simulink library "rtwvariantslib"  (Simulink 7.6)
settings: Solver=FixedStepDiscrete  StartTime=0.0  StopTime=10.0  RelTol=1e-3
undefined symbols (not defined in the file or in its folder): Variant1, Variant2
libraries: rtwvariantslib x2
settings Model: Creator=The MathWorks Inc.

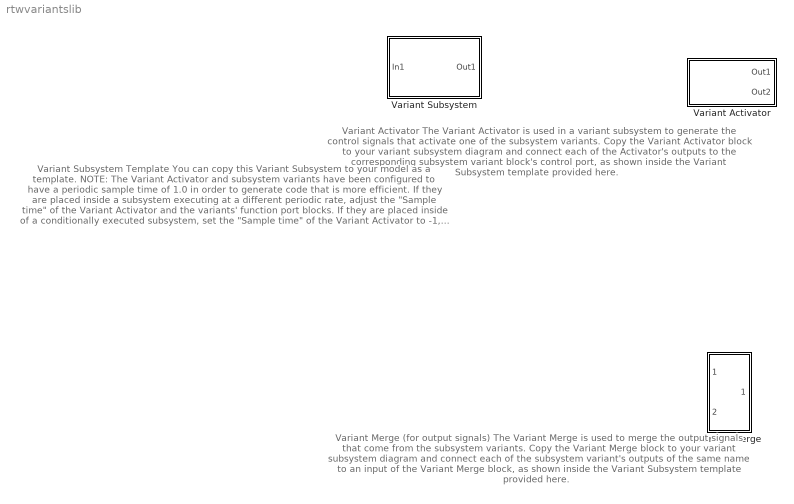
== system rtwvariantslib ==
  note: Variant Merge (for output signals)
      |
      | The Variant Merge
      | is used to merge
      | the output signals
      | that come from the
      | subsystem variants.
      |
      |
      | Copy the Variant Merge block to your
      | variant subsystem diagram and connect
      | each of the subsystem variant's outputs
      | of the same name to an input of
      | the Variant Merge block, as shown
      | inside the Variant Subsystem
      | template provided here.
  note: Variant Activator
      |
      | The Variant Activator
      | is used in a variant
      | subsystem to
      | generate the control
      | signals that activate
      | one of the subsystem
      | variants.
      |
      | Copy the Variant Activator block to your
      | variant subsystem diagram and connect
      | each of the Activator's outputs to
      | the corresponding subsystem
      | variant block's control port, as shown
      | inside the Variant Subsystem
      | template provided here.
  note: Variant Subsystem Template
      |
      | You can copy this
      | Variant Subsystem
      | to your model as a
      | template.
      |
      | NOTE: The Variant Activator and subsystem
      | variants have been configured to have a
      | periodic sample time of 1.0 in order to
      | generate code that is more efficient.
      | If they are placed inside a subsystem
      | executing at a different periodic rate,
      | adjust the "Sample time" of the Variant
      | Activator and the variants' function port
      | blocks.
      | If they are placed inside of a conditionally
      | executed subsystem, set the "Sample time"
      | of the Variant Activator to -1, and the
      | "Sample time type" of the variants' function
      | port blocks to "triggered".
  Variant Activator : Subsystem  mask(Variant Activator){sample_time=1, condition=Variant1,Variant2, gen_preproc_cond=on}
      mask prompts: sample_time "Sample time:"; condition "Variants (comma-separated list of Simulink.Variant objects):"; gen_preproc_cond "Generate preprocessor conditionals"
      mask help:
      | The Variant Activator is used to generate the control signals that activate one of the function-call subsystems.
      |
      | Enter the names of the Variant Objects in the Variants field as a comma-separated list. Variant objects are created in the base workspace and have conditions to determine which variant is active. For example:
      | >>  Variant1 = Simulink.Variant('A==1')
      | >>  Variant2 = Simulink.Variant('A==2')
      | Variant1 is active when A is equal to 1 and Variant2 is active when A is equal to 2. Only one Variant Object can be active during simulation.
      mask init:
      | rtwprivate('VariantActivatorInitializationCommands',condition);
      mask Display: port_label('output',1,'Variant1'); port_label('output',2,'Variant2');
  Variant Merge : Subsystem  mask(Variant Merge){numInputs=2}
      mask prompts: numInputs "Number of Inputs:"
      mask help: This block is used in a variant subsystem to merge the corresponding outputs from subsystem variant blocks.
      mask init:
      | rtwprivate('VariantMergeInitializationCommands',numInputs);
      mask Display: disp('Variant\nMerge')
  Variant Subsystem : Subsystem
      settings: CopyFcn=|
      | set_param(gcb, 'LinkStatus', 'none');
      | set_param(gcb, 'CopyFcn', '');

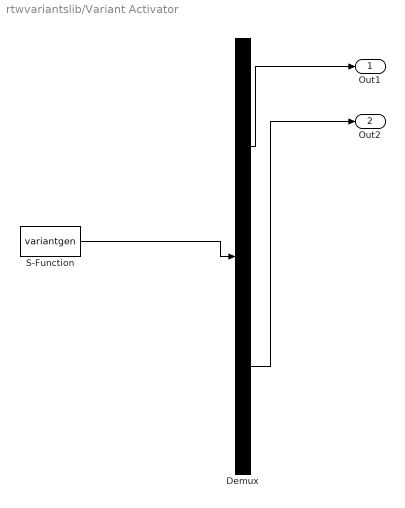
== system rtwvariantslib/Variant Activator ==
  Demux : Demux  Outputs=2
  S-Function : S-Function  FunctionName=variantgen  Parameters=sample_time,1,condition,gen_preproc_cond  EnableBusSupport=off
  Out1 : Outport
  Out2 : Outport  Port=2
  wires:
  Demux/1 -> Out1/1
  S-Function/1 -> Demux/1
  Demux/2 -> Out2/1

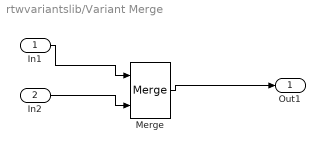
== system rtwvariantslib/Variant Merge ==
  In1 : Inport
  In2 : Inport  Port=2
  Merge : Merge
  Out1 : Outport
  wires:
  In2/1 -> Merge/2
  In1/1 -> Merge/1
  Merge/1 -> Out1/1

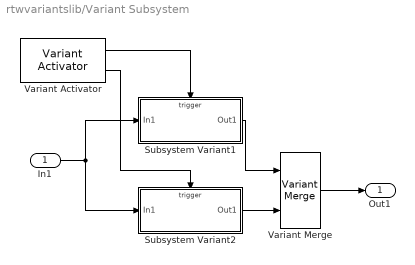
== system rtwvariantslib/Variant Subsystem ==
  In1 : Inport
  Subsystem Variant1 : Subsystem  TreatAsAtomicUnit=on
      settings: CopyFcn=|
      | set_param(gcb, 'LinkStatus', 'none');
      | set_param(gcb, 'CopyFcn', '');
  Subsystem Variant2 : Subsystem  TreatAsAtomicUnit=on
      settings: CopyFcn=|
      | set_param(gcb, 'LinkStatus', 'none');
      | set_param(gcb, 'CopyFcn', '');
  Variant Activator : rtwvariantslib/Variant Activator  SystemSampleTime=-1  sample_time=1  condition=Variant1,Variant2  gen_preproc_cond=on
  Variant Merge : rtwvariantslib/Variant Merge  SystemSampleTime=-1  numInputs=2
  Out1 : Outport
  wires:
  Variant Activator/1 -> Subsystem Variant1/Trigger
  Variant Activator/2 -> Subsystem Variant2/Trigger
  Subsystem Variant1/1(Out1) -> Variant Merge/1
  Subsystem Variant2/1(Out1) -> Variant Merge/2
  Variant Merge/1 -> Out1/1
  In1/1 -> Subsystem Variant1/1(In1), Subsystem Variant2/1(In1)

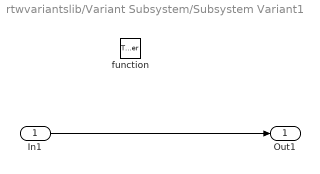
== system rtwvariantslib/Variant Subsystem/Subsystem Variant1 ==
  In1 : Inport
  function : TriggerPort  TriggerType=function-call  SampleTimeType=periodic
  Out1 : Outport
  wires:
  In1/1 -> Out1/1

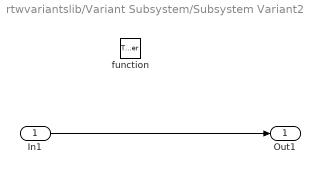
== system rtwvariantslib/Variant Subsystem/Subsystem Variant2 ==
  In1 : Inport
  function : TriggerPort  TriggerType=function-call  SampleTimeType=periodic
  Out1 : Outport
  wires:
  In1/1 -> Out1/1
